simulink model "Test_Word_Multiplexer_16_to_1"  (Simulink 8.7)
settings: Solver=ode45  StartTime=0.0  StopTime=len  RelTol=1e-3
libraries: Miscellaneous x17, commutil2 x1, Word_Multiplexers_Lib x1
settings Model: Creator=N  LastModifiedBy=Jozko Mrkvicka
settings DataIOCC: LimitDataPoints=off
settings DebuggingCC: UnderspecifiedInitializationDetection=Simplified  MergeDetectMultiDrivingBlocksExec=error
settings HardwareCC: ProdBitPerPointer=64  ProdLargestAtomicFloat=Float  ProdIntDivRoundTo=Zero  ProdEndianess=LittleEndian  ProdHWDeviceType=Intel->x86-64 (Windows64)
settings ModelReferenceCC: PropagateSignalLabelsOutOfModel=on

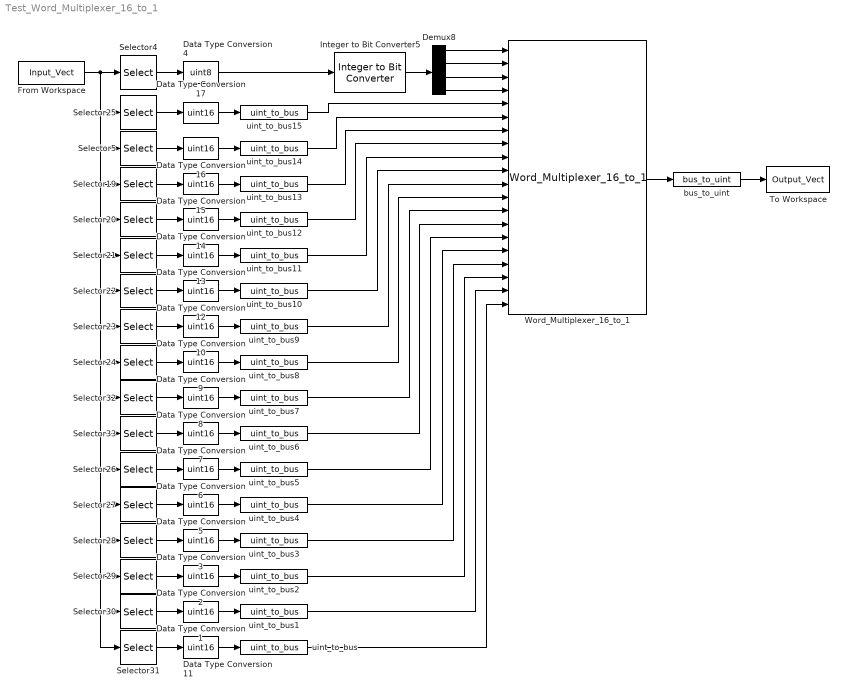
== system Test_Word_Multiplexer_16_to_1 ==
  Data Type Conversion{1..3,5..17} (16 alike) : DataTypeConversion  OutDataTypeStr=uint16
  Data Type Conversion4 : DataTypeConversion  OutDataTypeStr=uint8
  Demux8 : Demux
  From Workspace : FromWorkspace  VariableName=Input_Vect  SampleTime=1  Interpolate=off  OutputAfterFinalValue=Holding final value
  Integer to Bit Converter5 : commutil2/Integer to Bit Converter  nbits=4  signedInputValues=Unsigned  bitOrder=MSB first  outDtype=boolean
  Selector19 : Selector  IndexMode=Zero-based  InputPortWidth=17  IndexOptions=Index vector (dialog)  Indices=3  OutputSizes=1
  Selector20 : Selector  IndexMode=Zero-based  InputPortWidth=17  IndexOptions=Index vector (dialog)  Indices=4  OutputSizes=1
  Selector21 : Selector  IndexMode=Zero-based  InputPortWidth=17  IndexOptions=Index vector (dialog)  Indices=5  OutputSizes=1
  Selector22 : Selector  IndexMode=Zero-based  InputPortWidth=17  IndexOptions=Index vector (dialog)  Indices=6  OutputSizes=1
  Selector23 : Selector  IndexMode=Zero-based  InputPortWidth=17  IndexOptions=Index vector (dialog)  Indices=7  OutputSizes=1
  Selector24 : Selector  IndexMode=Zero-based  InputPortWidth=17  IndexOptions=Index vector (dialog)  Indices=8  OutputSizes=1
  Selector25 : Selector  IndexMode=Zero-based  InputPortWidth=17  IndexOptions=Index vector (dialog)  Indices=1  OutputSizes=1
  Selector26 : Selector  IndexMode=Zero-based  InputPortWidth=17  IndexOptions=Index vector (dialog)  Indices=11  OutputSizes=1
  Selector27 : Selector  IndexMode=Zero-based  InputPortWidth=17  IndexOptions=Index vector (dialog)  Indices=12  OutputSizes=1
  Selector28 : Selector  IndexMode=Zero-based  InputPortWidth=17  IndexOptions=Index vector (dialog)  Indices=13  OutputSizes=1
  Selector29 : Selector  IndexMode=Zero-based  InputPortWidth=17  IndexOptions=Index vector (dialog)  Indices=14  OutputSizes=1
  Selector30 : Selector  IndexMode=Zero-based  InputPortWidth=17  IndexOptions=Index vector (dialog)  Indices=15  OutputSizes=1
  Selector31 : Selector  IndexMode=Zero-based  InputPortWidth=17  IndexOptions=Index vector (dialog)  Indices=16  OutputSizes=1
  Selector32 : Selector  IndexMode=Zero-based  InputPortWidth=17  IndexOptions=Index vector (dialog)  Indices=9  OutputSizes=1
  Selector33 : Selector  IndexMode=Zero-based  InputPortWidth=17  IndexOptions=Index vector (dialog)  Indices=10  OutputSizes=1
  Selector4 : Selector  IndexMode=Zero-based  InputPortWidth=17  SampleTime=1  IndexOptions=Index vector (dialog)  Indices=0  OutputSizes=1
  Selector5 : Selector  IndexMode=Zero-based  InputPortWidth=17  IndexOptions=Index vector (dialog)  Indices=2  OutputSizes=1
  To Workspace : ToWorkspace  VariableName=Output_Vect  SampleTime=1
  Word_Multiplexer_16_to_1 : Word_Multiplexers_Lib/Word_Multiplexers_Lib/Word_Multiplexer_16_to_1
  bus_to_uint : Miscellaneous/bus_to_uint
  uint_to_bus{,1..15} (16 alike) : Miscellaneous/uint_to_bus
  wires:
  Integer to Bit Converter5/1 -> Demux8/1
  Word_Multiplexer_16_to_1/1 -> bus_to_uint/1
  Demux8/1 -> Word_Multiplexer_16_to_1/1
  Demux8/3 -> Word_Multiplexer_16_to_1/3
  Demux8/2 -> Word_Multiplexer_16_to_1/2
  Demux8/4 -> Word_Multiplexer_16_to_1/4
  Selector4/1 -> Data Type Conversion4/1
  Data Type Conversion4/1 -> Integer to Bit Converter5/1
  From Workspace/1 -> Selector5/1, Selector19/1, Selector20/1, Selector21/1, Selector22/1, Selector23/1, Selector32/1, Selector33/1, Selector26/1, Selector27/1, Selector28/1, Selector29/1, Selector30/1, Selector31/1, Selector24/1, Selector25/1, Selector4/1
  Selector25/1 -> Data Type Conversion17/1
  Selector5/1 -> Data Type Conversion16/1
  Selector19/1 -> Data Type Conversion15/1
  Selector20/1 -> Data Type Conversion14/1
  Selector21/1 -> Data Type Conversion13/1
  Selector22/1 -> Data Type Conversion12/1
  Selector23/1 -> Data Type Conversion10/1
  Selector24/1 -> Data Type Conversion9/1
  Selector32/1 -> Data Type Conversion8/1
  Selector33/1 -> Data Type Conversion7/1
  Selector26/1 -> Data Type Conversion6/1
  Selector27/1 -> Data Type Conversion5/1
  Selector28/1 -> Data Type Conversion3/1
  Selector29/1 -> Data Type Conversion2/1
  Selector30/1 -> Data Type Conversion1/1
  Selector31/1 -> Data Type Conversion11/1
  Data Type Conversion17/1 -> uint_to_bus15/1
  Data Type Conversion16/1 -> uint_to_bus14/1
  Data Type Conversion15/1 -> uint_to_bus13/1
  Data Type Conversion14/1 -> uint_to_bus12/1
  Data Type Conversion13/1 -> uint_to_bus11/1
  Data Type Conversion12/1 -> uint_to_bus10/1
  Data Type Conversion10/1 -> uint_to_bus9/1
  Data Type Conversion9/1 -> uint_to_bus8/1
  Data Type Conversion8/1 -> uint_to_bus7/1
  Data Type Conversion7/1 -> uint_to_bus6/1
  Data Type Conversion6/1 -> uint_to_bus5/1
  Data Type Conversion5/1 -> uint_to_bus4/1
  Data Type Conversion3/1 -> uint_to_bus3/1
  Data Type Conversion2/1 -> uint_to_bus2/1
  Data Type Conversion1/1 -> uint_to_bus1/1
  Data Type Conversion11/1 -> uint_to_bus/1
  bus_to_uint/1 -> To Workspace/1
  uint_to_bus/1 -> Word_Multiplexer_16_to_1/20
  uint_to_bus1/1 -> Word_Multiplexer_16_to_1/19
  uint_to_bus2/1 -> Word_Multiplexer_16_to_1/18
  uint_to_bus3/1 -> Word_Multiplexer_16_to_1/17
  uint_to_bus4/1 -> Word_Multiplexer_16_to_1/16
  uint_to_bus5/1 -> Word_Multiplexer_16_to_1/15
  uint_to_bus6/1 -> Word_Multiplexer_16_to_1/14
  uint_to_bus7/1 -> Word_Multiplexer_16_to_1/13
  uint_to_bus8/1 -> Word_Multiplexer_16_to_1/12
  uint_to_bus9/1 -> Word_Multiplexer_16_to_1/11
  uint_to_bus10/1 -> Word_Multiplexer_16_to_1/10
  uint_to_bus11/1 -> Word_Multiplexer_16_to_1/9
  uint_to_bus12/1 -> Word_Multiplexer_16_to_1/8
  uint_to_bus13/1 -> Word_Multiplexer_16_to_1/7
  uint_to_bus14/1 -> Word_Multiplexer_16_to_1/6
  uint_to_bus15/1 -> Word_Multiplexer_16_to_1/5
